simulink model "SampleTimeMath"  (R2017b)
settings: Solver=FixedStepDiscrete  StartTime=0.0  StopTime=10.0  FixedStep=0.200000  RelTol=1e-3  EnableMultiTasking=on
settings Model: Creator=hbourbou  LastModifiedBy=hbourbou
settings DataIOCC: LimitDataPoints=on  SaveFormat=StructureWithTime
settings OptimizationCC: LifeSpan=inf
settings DebuggingCC: SFUnexpectedBacktrackingDiag=warning  SFNoUnconditionalDefaultTransitionDiag=warning  SFExecutionAtInitializationDiag=none
settings HardwareCC: ProdBitPerSizeT=32  ProdBitPerPtrDiffT=32  ProdWordSize=32  ProdHWDeviceType=Specified
settings ModelReferenceCC: PropagateSignalLabelsOutOfModel=off
settings CodeAppCC: StateflowObjectComments=on
settings GRTTargetCC: TargetLangStandard=C89/C90 (ANSI)
settings ConfigComp: CovMetricSettings=dw  CovHtmlReporting=on  CovSaveCumulativeToWorkspaceVar=on  CovSaveSingleToWorkspaceVar=on  CovExternalEMLEnable=off

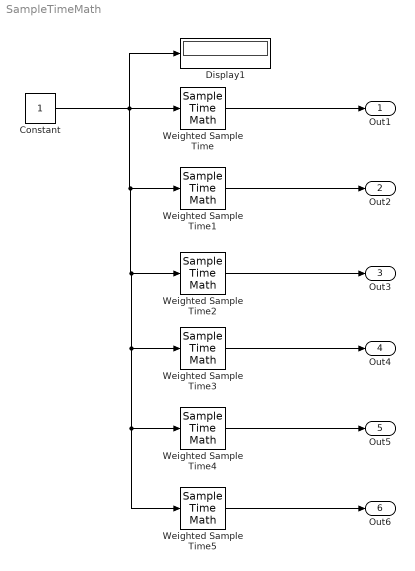
== system SampleTimeMath ==
  Constant : Constant
  Display1 : Display
  Weighted Sample Time : SampleTimeMath  weightValue=2
  Weighted Sample Time1 : SampleTimeMath  TsampMathOp=-  weightValue=2
  Weighted Sample Time2 : SampleTimeMath  TsampMathOp=*  weightValue=2
  Weighted Sample Time3 : SampleTimeMath  TsampMathOp=/  weightValue=2
  Weighted Sample Time4 : SampleTimeMath  TsampMathOp=Ts Only  weightValue=2
  Weighted Sample Time5 : SampleTimeMath  TsampMathOp=1/Ts Only  weightValue=2
  Out1 : Outport
  Out2 : Outport  Port=2
  Out3 : Outport  Port=3
  Out4 : Outport  Port=4
  Out5 : Outport  Port=5
  Out6 : Outport  Port=6
  wires:
  Constant/1 -> Weighted Sample Time5/1, Weighted Sample Time4/1, Weighted Sample Time3/1, Weighted Sample Time2/1, Weighted Sample Time1/1, Display1/1, Weighted Sample Time/1
  Weighted Sample Time/1 -> Out1/1
  Weighted Sample Time1/1 -> Out2/1
  Weighted Sample Time2/1 -> Out3/1
  Weighted Sample Time3/1 -> Out4/1
  Weighted Sample Time4/1 -> Out5/1
  Weighted Sample Time5/1 -> Out6/1
